simulink model "hgv_q_monitor"  (R2023b)
settings: Solver=FixedStepDiscrete  StartTime=0.0  StopTime=0  FixedStep=1  RelTol=1e-3
settings Model: Creator=luoman  LastModifiedBy=luoman

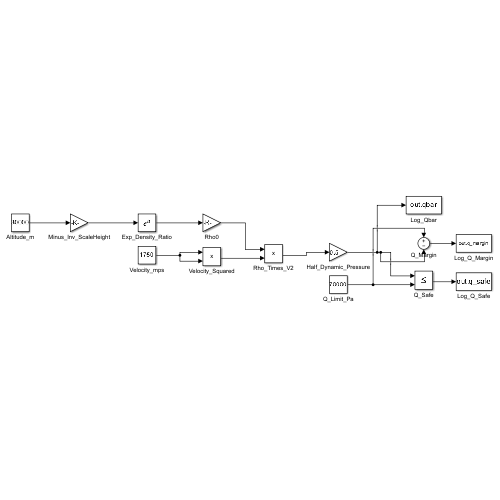
[thumbnail: Simulink's stored preview of the top-level diagram]
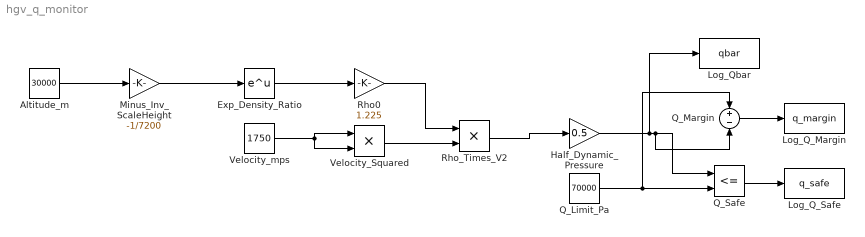
== system hgv_q_monitor ==
  Altitude_m : Constant  Value=30000
  Exp_Density_Ratio : Math  SignedPower=on  RndMeth=Zero
  Half_Dynamic_Pressure : Gain  Gain=0.5
  Log_Q_Margin : ToWorkspace  VariableName=q_margin  SampleTime=-1
  Log_Q_Safe : ToWorkspace  VariableName=q_safe  SampleTime=-1
  Log_Qbar : ToWorkspace  VariableName=qbar  SampleTime=-1
  Minus_Inv_ScaleHeight : Gain  Gain=-1/7200
  Q_Limit_Pa : Constant  Value=70000
  Q_Margin : Sum  Inputs=+-
  Q_Safe : RelationalOperator  Operator=<=  OutDataTypeStr=boolean  InputSameDT=off
  Rho0 : Gain  Gain=1.225
  Rho_Times_V2 : Product  Inputs=**
  Velocity_Squared : Product  Inputs=**
  Velocity_mps : Constant  Value=1750
  wires:
  Q_Safe/1 -> Log_Q_Safe/1
  Q_Margin/1 -> Log_Q_Margin/1
  Half_Dynamic_Pressure/1 -> Q_Safe/1, Q_Margin/2, Log_Qbar/1
  Q_Limit_Pa/1 -> Q_Safe/2, Q_Margin/1
  Rho_Times_V2/1 -> Half_Dynamic_Pressure/1
  Velocity_Squared/1 -> Rho_Times_V2/2
  Rho0/1 -> Rho_Times_V2/1
  Velocity_mps/1 -> Velocity_Squared/2, Velocity_Squared/1
  Exp_Density_Ratio/1 -> Rho0/1
  Minus_Inv_ScaleHeight/1 -> Exp_Density_Ratio/1
  Altitude_m/1 -> Minus_Inv_ScaleHeight/1
